simulink model "termin7simulink"  (R2022b)
settings: Solver=VariableStepAuto  StartTime=0.0  StopTime=t_simulation  MaxStep=0.1  RelTol=1e-3
values from neighbouring files (symbols this model uses):
  Cvp = cp * rop * Vp    (= 90000)    [matlablab12.m]    (also in zajeciatermin7matalb.m)
  Cvw = cp * rop * Vw    (= 150000)    [matlablab12.m]    (also in zajeciatermin7matalb.m)
  dTzad = 3    [matlablab12.m]    (also in zajeciatermin7matalb.m = 5)
  dTzew = 3    [matlablab12.m]    (also in zajeciatermin7matalb.m = 0)
  K = 0.003    [zajeciatermin7matalb.m]
  Kcp = (qgN*a*(TwewN-TpN))/((TwewN * (1 + a) - TzewN - a*TpN)  * (TpN - TzewN))    (= 19.6078431373)    [matlablab12.m]    (also in zajeciatermin7matalb.m)
  Kcw = qgN/(TwewN * (1 + a) - TzewN - a * TpN)    (= 235.294117647)    [matlablab12.m]    (also in zajeciatermin7matalb.m)
  Kcwp = a*qgN/(TwewN*(1+a) -TzewN - a*TpN)    (= 58.8235294118)    [matlablab12.m]    (also in zajeciatermin7matalb.m)
  Ki = 0.0019157    [matlablab12.m]    (also in zajeciatermin7matalb.m = 0.000435217826522)
  KiTunerModel = KiTunerModeloop(i)    [zajeciatermin7matalb.m]
  KiTunerObjekt = 0.42897    [zajeciatermin7matalb.m]
  Kp = 0.058968    [matlablab12.m]    (also in zajeciatermin7matalb.m = 369.565217391)
  KpTunerModel = KpTunerModelloop(i)    [zajeciatermin7matalb.m]
  KpTunerObjekt = 544.8728    [zajeciatermin7matalb.m]
  qg0 = Twew0*(Kcw+Kcwp)-Tp0*Kcwp-Kcw*((Tp0*(Kcp+Kcwp)-Twew0*Kcwp)/Kcp)    (= 10000)    [matlablab12.m]    (also in zajeciatermin7matalb.m)
  t0 = 10    [matlablab12.m]    (also in zajeciatermin7matalb.m = 5000)
  T0TpDP = 690    [zajeciatermin7matalb.m]
  Tp0 = ((Kcw + Kcwp)*Kcp*Tzew0 + Kcwp*(qg0 + Kcw*Tzew0))/(Kcw*(Kcwp + Kcp) + Kcwp*Kcp)    (= 10)    [matlablab12.m]    (also in zajeciatermin7matalb.m)
  trasport_delayDP = 689    [zajeciatermin7matalb.m]
  Twew0 = (qg0*(Kcwp + Kcp) + Tzew0*(Kcw*Kcwp + Kcw * Kcp + Kcwp * Kcp))/(Kcw*(Kcwp + Kcp) + Kcwp * Kcp)    (= 20)    [matlablab12.m]    (also in zajeciatermin7matalb.m)
  Tzad = TpN    (= 10)    [matlablab12.m]    (also in zajeciatermin7matalb.m)
  Tzew0 = TzewN    (= -20)    [matlablab12.m]    (also in zajeciatermin7matalb.m)
libraries: slpidlib x2
settings Model: Creator=huber  LastModifiedBy=huber
settings DataIOCC: ReturnWorkspaceOutputs=off

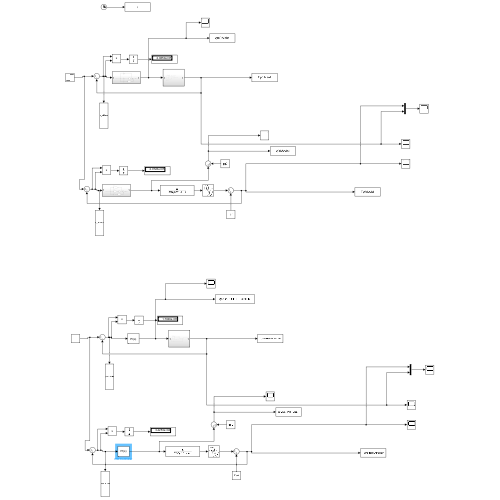
[thumbnail: Simulink's stored preview of the top-level diagram]
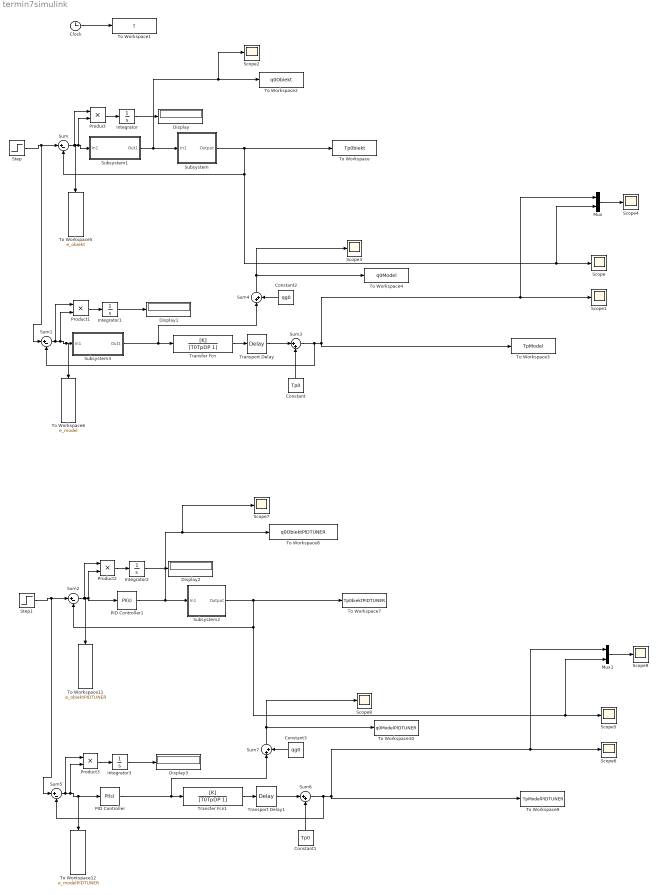
== system termin7simulink ==
  Clock : Clock
  Constant : Constant  Value=Tp0
  Constant1 : Constant  Value=Tp0
  Constant2 : Constant  Value=qg0
  Constant3 : Constant  Value=qg0
  Display{,1..3} (4 alike) : Display
      settings: Format=short_e
  Integrator{,1..3} (4 alike) : Integrator
  Mux : Mux  Inputs=2
  Mux1 : Mux  Inputs=2
  PID Controller : slpidlib/PID Controller  Controller=PI  Form=Parallel  TimeDomain=Continuous-time  UseExternalTs=off  SampleTime=-1  IntegratorMethod=Forward Euler  FilterMethod=Forward Euler  ControllerParametersSource=internal  P=KpTunerModel  I=KiTunerModel  UseKiTs=off  D=0  N=100  UseFilter=on  TunerSelectOption=Transfer Function Based (PID Tuner App)  InitialConditionSource=internal  InitialConditionForIntegrator=0  InitialConditionForFilter=0  DifferentiatorICPrevScaledInput=0  ExternalReset=none  TrackingMode=off  Kt=1  LimitOutput=off  SatLimitsSource=internal  UpperSaturationLimit=inf  LowerSaturationLimit=-inf  LinearizeAsGain=on  AntiWindupMode=none  Kb=1  LimitIntegrator=off  UpperIntegratorSaturationLimit=inf  LowerIntegratorSaturationLimit=-inf  POutMin=[]  POutMax=[]  IOutMin=[]  IOutMax=[]  DOutMin=[]  DOutMax=[]  NOutMin=[]  NOutMax=[]  SumOutMin=[]  SumOutMax=[]  SaturationOutMin=[]  SaturationOutMax=[]  PParamMin=[]  PParamMax=[]  IParamMin=[]  IParamMax=[]  DParamMin=[]  DParamMax=[]  NParamMin=[]  NParamMax=[]  KbParamMin=[]  KbParamMax=[]  KtParamMin=[]  KtParamMax=[]  KbOutMin=[]  KbOutMax=[]  KtOutMin=[]  KtOutMax=[]  IntegratorOutMin=[]  IntegratorOutMax=[]  FilterOutMin=[]  FilterOutMax=[]  SumI1OutMin=[]  SumI1OutMax=[]  SumI2OutMin=[]  SumI2OutMax=[]  SumI3OutMin=[]  SumI3OutMax=[]  SumI4OutMin=[]  SumI4OutMax=[]  SumDOutMin=[]  SumDOutMax=[]  DifferentiatorOutMin=[]  DifferentiatorOutMax=[]  FilterDiffOutCoefMin=[]  FilterDiffOutCoefMax=[]  ReciprocalOutMin=[]  ReciprocalOutMax=[]  SumDenOutMin=[]  SumDenOutMax=[]  SumNumOutMin=[]  SumNumOutMax=[]  DivideOutMin=[]  DivideOutMax=[]  UdiffTsProdOutMin=[]  UdiffTsProdOutMax=[]  NTsProdOutMin=[]  NTsProdOutMax=[]  UintegralTsProdOutMin=[]  UintegralTsProdOutMax=[]  UngainTsProdOutMin=[]  UngainTsProdOutMax=[]  ClampingZeroOutDataTypeStr=Inherit: Inherit via back propagation  ClampingZeroOutMin=[]  ClampingZeroOutMax=[]  FilterDenConstantOutDataTypeStr=Inherit: Inherit via back propagation  FilterDenConstantOutMin=[]  FilterDenConstantOutMax=[]  PCopyOutDataTypeStr=Inherit: Inherit via back propagation  PCopyOutMin=[]  PCopyOutMax=[]  NCopyOutDataTypeStr=Inherit: Inherit via back propagation  NCopyOutMin=[]  NCopyOutMax=[]  IntegratorContinuousStateAttributes=''  IntegratorStateMustResolveToSignalObject=off  IntegratorRTWStateStorageClass=Auto  FilterContinuousStateAttributes=''  FilterStateMustResolveToSignalObject=off  FilterRTWStateStorageClass=Auto  ParallelPVariant=InternalParameters  IdealPVariant=Disabled  IVariant=InternalParameters  DVariant=Disabled  IntegratorVariant=Continuous  SatVariant=Disabled  AWVariant=Passthrough  PCopyVariant=Disabled  TRVariant=Disabled  FdbkBlocksVariant=Forward  IdealPFdbkVariant=Disabled  SatFdbkVariant=Disabled  DerivativeFilterVariant=Disabled  NVariant=Disabled  NCopyVariant=Disabled_SignalSpec  FilterICVariant=Disabled  IntegratorICVariant=InternalICs  ExternalResetVariant=Disabled  TRSumVariant=Passthrough  SumFdbkVariant=Disabled  SumVariant=Sum_PI  TsampFilterVariant=InternalTs  TsampNgainVariant=Passthrough  TsampIntegralVariant=Passthrough  ExternalSaturationOutDataTypeStr=Inherit: Same as second input
  PID Controller1 : slpidlib/PID Controller  Controller=PI  Form=Parallel  TimeDomain=Continuous-time  UseExternalTs=off  SampleTime=-1  IntegratorMethod=Forward Euler  FilterMethod=Forward Euler  ControllerParametersSource=internal  P=KpTunerObjekt  I=KiTunerObjekt  UseKiTs=off  D=0  N=100  UseFilter=on  TunerSelectOption=Transfer Function Based (PID Tuner App)  InitialConditionSource=internal  InitialConditionForIntegrator=0  InitialConditionForFilter=0  DifferentiatorICPrevScaledInput=0  ExternalReset=none  TrackingMode=off  Kt=1  LimitOutput=off  SatLimitsSource=internal  UpperSaturationLimit=inf  LowerSaturationLimit=-inf  LinearizeAsGain=on  AntiWindupMode=none  Kb=1  LimitIntegrator=off  UpperIntegratorSaturationLimit=inf  LowerIntegratorSaturationLimit=-inf  POutMin=[]  POutMax=[]  IOutMin=[]  IOutMax=[]  DOutMin=[]  DOutMax=[]  NOutMin=[]  NOutMax=[]  SumOutMin=[]  SumOutMax=[]  SaturationOutMin=[]  SaturationOutMax=[]  PParamMin=[]  PParamMax=[]  IParamMin=[]  IParamMax=[]  DParamMin=[]  DParamMax=[]  NParamMin=[]  NParamMax=[]  KbParamMin=[]  KbParamMax=[]  KtParamMin=[]  KtParamMax=[]  KbOutMin=[]  KbOutMax=[]  KtOutMin=[]  KtOutMax=[]  IntegratorOutMin=[]  IntegratorOutMax=[]  FilterOutMin=[]  FilterOutMax=[]  SumI1OutMin=[]  SumI1OutMax=[]  SumI2OutMin=[]  SumI2OutMax=[]  SumI3OutMin=[]  SumI3OutMax=[]  SumI4OutMin=[]  SumI4OutMax=[]  SumDOutMin=[]  SumDOutMax=[]  DifferentiatorOutMin=[]  DifferentiatorOutMax=[]  FilterDiffOutCoefMin=[]  FilterDiffOutCoefMax=[]  ReciprocalOutMin=[]  ReciprocalOutMax=[]  SumDenOutMin=[]  SumDenOutMax=[]  SumNumOutMin=[]  SumNumOutMax=[]  DivideOutMin=[]  DivideOutMax=[]  UdiffTsProdOutMin=[]  UdiffTsProdOutMax=[]  NTsProdOutMin=[]  NTsProdOutMax=[]  UintegralTsProdOutMin=[]  UintegralTsProdOutMax=[]  UngainTsProdOutMin=[]  UngainTsProdOutMax=[]  ClampingZeroOutDataTypeStr=Inherit: Inherit via back propagation  ClampingZeroOutMin=[]  ClampingZeroOutMax=[]  FilterDenConstantOutDataTypeStr=Inherit: Inherit via back propagation  FilterDenConstantOutMin=[]  FilterDenConstantOutMax=[]  PCopyOutDataTypeStr=Inherit: Inherit via back propagation  PCopyOutMin=[]  PCopyOutMax=[]  NCopyOutDataTypeStr=Inherit: Inherit via back propagation  NCopyOutMin=[]  NCopyOutMax=[]  IntegratorContinuousStateAttributes=''  IntegratorStateMustResolveToSignalObject=off  IntegratorRTWStateStorageClass=Auto  FilterContinuousStateAttributes=''  FilterStateMustResolveToSignalObject=off  FilterRTWStateStorageClass=Auto  ParallelPVariant=InternalParameters  IdealPVariant=Disabled  IVariant=InternalParameters  DVariant=Disabled  IntegratorVariant=Continuous  SatVariant=Disabled  AWVariant=Passthrough  PCopyVariant=Disabled  TRVariant=Disabled  FdbkBlocksVariant=Forward  IdealPFdbkVariant=Disabled  SatFdbkVariant=Disabled  DerivativeFilterVariant=Disabled  NVariant=Disabled  NCopyVariant=Disabled_SignalSpec  FilterICVariant=Disabled  IntegratorICVariant=InternalICs  ExternalResetVariant=Disabled  TRSumVariant=Passthrough  SumFdbkVariant=Disabled  SumVariant=Sum_PI  TsampFilterVariant=InternalTs  TsampNgainVariant=Passthrough  TsampIntegralVariant=Passthrough  ExternalSaturationOutDataTypeStr=Inherit: Same as second input
  Product{,1..3} (4 alike) : Product
  Scope{,1..9} (10 alike) : Scope
  Step : Step  Time=t0  Before=Tzad  After=Tzad + dTzad  SampleTime=0
  Step1 : Step  Time=t0  Before=Tzad  After=Tzad + dTzad  SampleTime=0
  Subsystem : Subsystem
  Subsystem1 : Subsystem
  Subsystem2 : Subsystem
  Subsystem3 : Subsystem
  Sum{,1..2,5} (4 alike) : Sum  Inputs=|+-
  Sum{3..4,6..7} (4 alike) : Sum  Inputs=|++
  To Workspace : ToWorkspace  VariableName=Tp0biekt  SampleTime=-1
  To Workspace1 : ToWorkspace  VariableName=t  SampleTime=-1
  To Workspace10 : ToWorkspace  VariableName=q0ModelPIDTUNER  SampleTime=-1
  To Workspace11 : ToWorkspace  VariableName=e_obiektPIDTUNER  SampleTime=-1
  To Workspace12 : ToWorkspace  VariableName=e_modelPIDTUNER  SampleTime=-1
  To Workspace2 : ToWorkspace  VariableName=q0Obiekt  SampleTime=-1
  To Workspace3 : ToWorkspace  VariableName=TpModel  SampleTime=-1
  To Workspace4 : ToWorkspace  VariableName=q0Model  SampleTime=-1
  To Workspace5 : ToWorkspace  VariableName=e_obiekt  SampleTime=-1
  To Workspace6 : ToWorkspace  VariableName=e_model  SampleTime=-1
  To Workspace7 : ToWorkspace  VariableName=Tp0biektPIDTUNER  SampleTime=-1
  To Workspace8 : ToWorkspace  VariableName=q0ObiektPIDTUNER  SampleTime=-1
  To Workspace9 : ToWorkspace  VariableName=TpModelPIDTUNER  SampleTime=-1
  Transfer Fcn : TransferFcn  Numerator=[K]  Denominator=[T0TpDP 1]
  Transfer Fcn1 : TransferFcn  Numerator=[K]  Denominator=[T0TpDP 1]
  Transport Delay : TransportDelay  DelayTime=trasport_delayDP  BufferSize=30000
  Transport Delay1 : TransportDelay  DelayTime=trasport_delayDP  BufferSize=30000
  wires:
  Constant/1 -> Sum3/2
  Constant2/1 -> Sum4/2
  Integrator1/1 -> Display1/1
  Subsystem3/1(Out1) -> Sum4/1, Transfer Fcn/1
  Subsystem/1(Output) -> Mux/2, Scope/1, Sum/2, To Workspace/1
  Step/1 -> Sum1/1, Sum/1
  Sum1/1 -> Product1/1, Product1/2, To Workspace6/1, Subsystem3/1(In1)
  Subsystem1/1(Out1) -> Scope2/1, To Workspace2/1, Subsystem/1(In1)
  Integrator/1 -> Display/1
  Product1/1 -> Integrator1/1
  Clock/1 -> To Workspace1/1
  Sum/1 -> Product/1, Product/2, Subsystem1/1(In1), To Workspace5/1
  Sum4/1 -> To Workspace4/1, Scope3/1
  Transfer Fcn/1 -> Transport Delay/1
  Sum3/1 -> Sum1/2, Mux/1, Scope1/1, To Workspace3/1
  Transport Delay/1 -> Sum3/1
  Product/1 -> Integrator/1
  Mux/1 -> Scope4/1
  Mux1/1 -> Scope9/1
  Subsystem2/1(Output) -> Mux1/2, Scope5/1, Sum2/2, To Workspace7/1
  Product2/1 -> Integrator2/1
  Transport Delay1/1 -> Sum6/1
  Product3/1 -> Integrator3/1
  Transfer Fcn1/1 -> Transport Delay1/1
  Sum2/1 -> Product2/1, Product2/2, PID Controller1/1, To Workspace11/1
  Constant3/1 -> Sum7/2
  Sum6/1 -> Sum5/2, Mux1/1, Scope6/1, To Workspace9/1
  Integrator2/1 -> Display2/1
  Sum7/1 -> To Workspace10/1, Scope8/1
  Step1/1 -> Sum5/1, Sum2/1
  Integrator3/1 -> Display3/1
  Sum5/1 -> Product3/1, Product3/2, PID Controller/1, To Workspace12/1
  Constant1/1 -> Sum6/2
  PID Controller/1 -> Sum7/1, Transfer Fcn1/1
  PID Controller1/1 -> Scope7/1, To Workspace8/1, Subsystem2/1(In1)

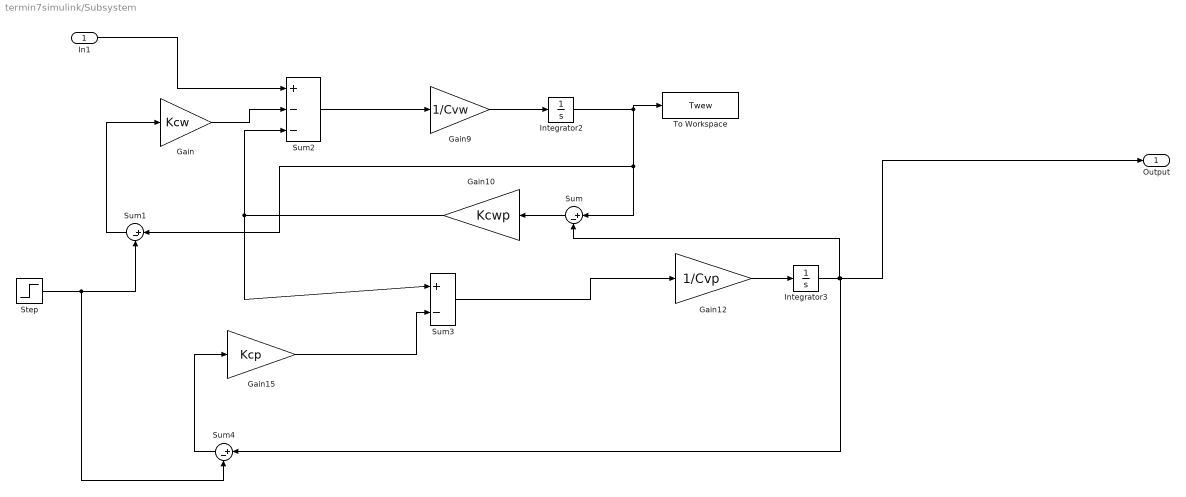
== system termin7simulink/Subsystem ==
  In1 : Inport
  Gain : Gain  Gain=Kcw
  Gain10 : Gain  Gain=Kcwp
  Gain12 : Gain  Gain=1/Cvp
  Gain15 : Gain  Gain=Kcp
  Gain9 : Gain  Gain=1/Cvw
  Integrator2 : Integrator  InitialCondition=Twew0
  Integrator3 : Integrator  InitialCondition=Tp0
  Step : Step  Time=t0  Before=Tzew0  After=Tzew0 + dTzew  SampleTime=0
  Sum{,1,3..4} (4 alike) : Sum  Inputs=|+-
  Sum2 : Sum  Inputs=+--
  To Workspace : ToWorkspace  VariableName=Twew  SampleTime=-1
  Output : Outport
  wires:
  Gain12/1 -> Integrator3/1
  Integrator2/1 -> To Workspace/1, Sum1/1, Sum/1
  Sum2/1 -> Gain9/1
  Gain9/1 -> Integrator2/1
  Gain10/1 -> Sum2/3, Sum3/1
  Integrator3/1 -> Output/1, Sum4/1, Sum/2
  Sum3/1 -> Gain12/1
  Gain15/1 -> Sum3/2
  In1/1 -> Sum2/1
  Step/1 -> Sum4/2, Sum1/2
  Gain/1 -> Sum2/2
  Sum1/1 -> Gain/1
  Sum/1 -> Gain10/1
  Sum4/1 -> Gain15/1

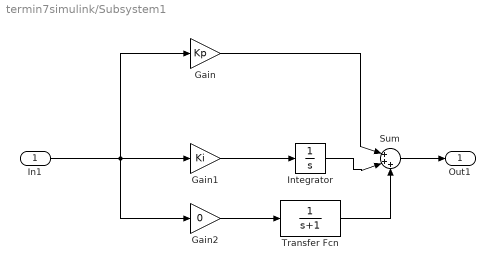
== system termin7simulink/Subsystem1 ==
  In1 : Inport
  Gain : Gain  Gain=Kp
  Gain1 : Gain  Gain=Ki
  Gain2 : Gain  Gain=0
  Integrator : Integrator  InitialCondition=qg0
  Sum : Sum  Inputs=|+++
  Transfer Fcn : TransferFcn  Denominator=[1 1]
  Out1 : Outport
  wires:
  In1/1 -> Gain2/1, Gain1/1, Gain/1
  Gain2/1 -> Transfer Fcn/1
  Gain/1 -> Sum/1
  Transfer Fcn/1 -> Sum/3
  Sum/1 -> Out1/1
  Gain1/1 -> Integrator/1
  Integrator/1 -> Sum/2

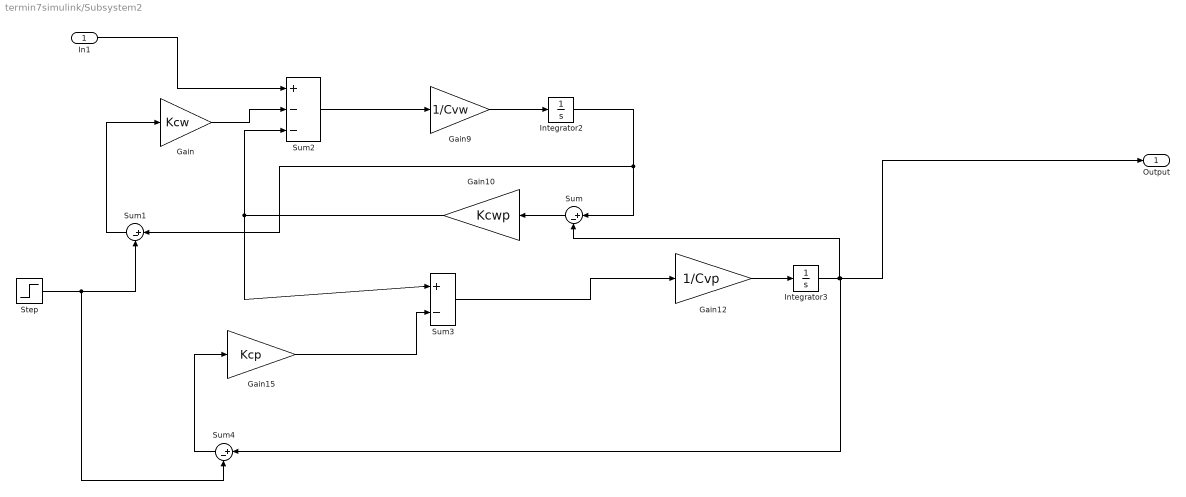
== system termin7simulink/Subsystem2 ==
  In1 : Inport
  Gain : Gain  Gain=Kcw
  Gain10 : Gain  Gain=Kcwp
  Gain12 : Gain  Gain=1/Cvp
  Gain15 : Gain  Gain=Kcp
  Gain9 : Gain  Gain=1/Cvw
  Integrator2 : Integrator  InitialCondition=Twew0
  Integrator3 : Integrator  InitialCondition=Tp0
  Step : Step  Time=t0  Before=Tzew0  After=Tzew0 + dTzew  SampleTime=0
  Sum{,1,3..4} (4 alike) : Sum  Inputs=|+-
  Sum2 : Sum  Inputs=+--
  Output : Outport
  wires:
  Gain12/1 -> Integrator3/1
  Integrator2/1 -> Sum1/1, Sum/1
  Sum2/1 -> Gain9/1
  Gain9/1 -> Integrator2/1
  Gain10/1 -> Sum2/3, Sum3/1
  Integrator3/1 -> Output/1, Sum4/1, Sum/2
  Sum3/1 -> Gain12/1
  Gain15/1 -> Sum3/2
  In1/1 -> Sum2/1
  Step/1 -> Sum4/2, Sum1/2
  Gain/1 -> Sum2/2
  Sum1/1 -> Gain/1
  Sum/1 -> Gain10/1
  Sum4/1 -> Gain15/1

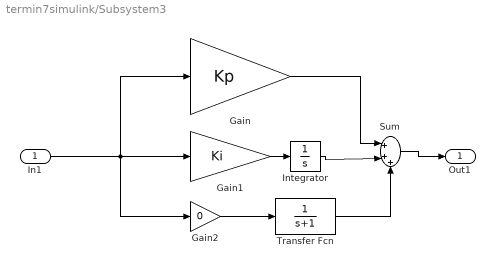
== system termin7simulink/Subsystem3 ==
  In1 : Inport
  Gain : Gain  Gain=Kp
  Gain1 : Gain  Gain=Ki
  Gain2 : Gain  Gain=0
  Integrator : Integrator
  Sum : Sum  Inputs=|+++
  Transfer Fcn : TransferFcn  Denominator=[1 1]
  Out1 : Outport
  wires:
  In1/1 -> Gain/1, Gain1/1, Gain2/1
  Gain/1 -> Sum/1
  Transfer Fcn/1 -> Sum/3
  Sum/1 -> Out1/1
  Gain2/1 -> Transfer Fcn/1
  Gain1/1 -> Integrator/1
  Integrator/1 -> Sum/2
